simulink model "NumberPlateV1"  (R2022a)
settings: Solver=VariableStepAuto  StartTime=0.0  StopTime=10.0  RelTol=1e-3
libraries: simulink x6
settings Model: Creator=riya4  LastModifiedBy=riya4

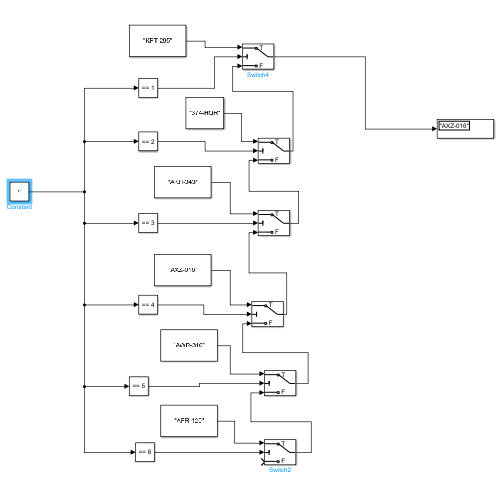
[thumbnail: Simulink's stored preview of the top-level diagram]
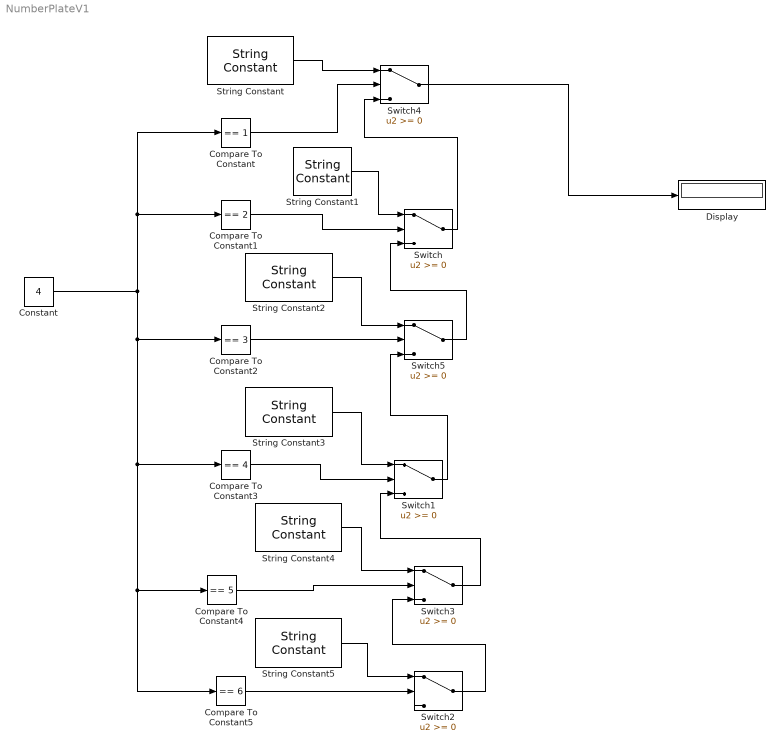
== system NumberPlateV1 ==
  Compare To Constant : simulink/Logic and Bit Operations/Compare To Constant  relop===  const=1  OutDataTypeStr=boolean
  Compare To Constant1 : simulink/Logic and Bit Operations/Compare To Constant  relop===  const=2  OutDataTypeStr=boolean
  Compare To Constant2 : simulink/Logic and Bit Operations/Compare To Constant  relop===  const=3  OutDataTypeStr=boolean
  Compare To Constant3 : simulink/Logic and Bit Operations/Compare To Constant  relop===  const=4  OutDataTypeStr=boolean
  Compare To Constant4 : simulink/Logic and Bit Operations/Compare To Constant  relop===  const=5  OutDataTypeStr=boolean
  Compare To Constant5 : simulink/Logic and Bit Operations/Compare To Constant  relop===  const=6  OutDataTypeStr=boolean
  Constant : Constant  Value=4
  Display : Display
  String Constant : StringConstant  String="\"KPT-295\""
  String Constant1 : StringConstant  String="\"374-HQR\""
  String Constant2 : StringConstant  String="\"AKH-343\""
  String Constant3 : StringConstant  String="\"AXZ-016\""
  String Constant4 : StringConstant  String="\"AWR-310\""
  String Constant5 : StringConstant  String="\"AFR-420\""
  Switch{,1..5} (6 alike) : Switch  SaturateOnIntegerOverflow=off  InputSameDT=off
  wires:
  Constant/1 -> Compare To Constant5/1, Compare To Constant4/1, Compare To Constant3/1, Compare To Constant2/1, Compare To Constant/1, Compare To Constant1/1
  Compare To Constant/1 -> Switch4/2
  Compare To Constant1/1 -> Switch/2
  Compare To Constant2/1 -> Switch5/2
  Compare To Constant3/1 -> Switch1/2
  Compare To Constant4/1 -> Switch3/2
  Compare To Constant5/1 -> Switch2/2
  String Constant/1 -> Switch4/1
  Switch/1 -> Switch4/3
  Switch5/1 -> Switch/3
  Switch1/1 -> Switch5/3
  Switch3/1 -> Switch1/3
  Switch2/1 -> Switch3/3
  String Constant1/1 -> Switch/1
  String Constant2/1 -> Switch5/1
  String Constant3/1 -> Switch1/1
  String Constant4/1 -> Switch3/1
  String Constant5/1 -> Switch2/1
  Switch4/1 -> Display/1
